simulink model "WindUp"  (R2018b)
settings: Solver=VariableStepAuto  StartTime=0.0  StopTime=100  RelTol=1e-3
settings Model: Creator=Alex  LastModifiedBy=Alex

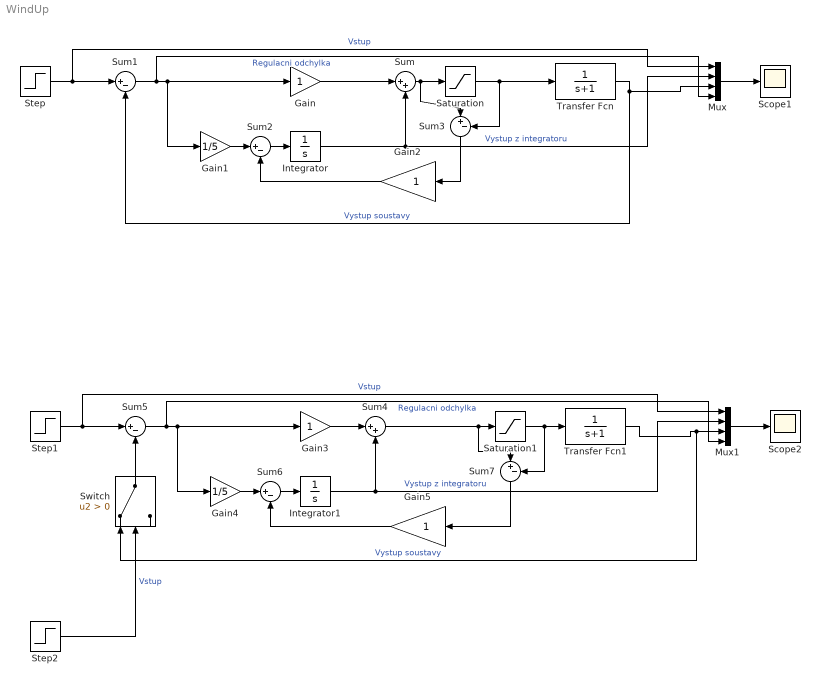
== system WindUp ==
  Gain{,2..3,5} (4 alike) : Gain
  Gain1 : Gain  Gain=1/5
  Gain4 : Gain  Gain=1/5
  Integrator : Integrator
  Integrator1 : Integrator
  Mux : Mux
  Mux1 : Mux
  Saturation : Saturate
  Saturation1 : Saturate
  Scope1 : Scope
  Scope2 : Scope
  Step : Step  Time=30  Before=1  After=0.2  SampleTime=0
  Step1 : Step  Time=30  Before=1  After=0.5  SampleTime=0
  Step2 : Step  Time=30  After=0.5  SampleTime=0
  Sum : Sum  Inputs=|++
  Sum{1..3,5..7} (6 alike) : Sum  Inputs=|+-
  Sum4 : Sum  Inputs=|++
  Switch : Switch  Criteria=u2 > Threshold
  Transfer Fcn : TransferFcn  Denominator=[1 1]
  Transfer Fcn1 : TransferFcn  Denominator=[1 1]
  wires:
  Integrator/1 -> Sum/2, Mux/2  "Vystup z integratoru"
  Gain/1 -> Sum/1
  Sum1/1 -> Mux/4, Gain1/1, Gain/1  "Regulacni odchylka"
  Step/1 -> Mux/1, Sum1/1  "Vstup"
  Sum/1 -> Sum3/1, Saturation/1
  Saturation/1 -> Sum3/2, Transfer Fcn/1
  Transfer Fcn/1 -> Mux/3, Sum1/2  "Vystup soustavy"
  Mux/1 -> Scope1/1
  Gain1/1 -> Sum2/1
  Sum2/1 -> Integrator/1
  Sum3/1 -> Gain2/1
  Gain2/1 -> Sum2/2
  Gain5/1 -> Sum6/2
  Gain3/1 -> Sum4/1
  Integrator1/1 -> Mux1/2, Sum4/2  "Vystup z integratoru"
  Transfer Fcn1/1 -> Switch/1, Mux1/3  "Vystup soustavy"
  Saturation1/1 -> Sum7/2, Transfer Fcn1/1
  Step1/1 -> Mux1/1, Sum5/1  "Vstup"
  Sum5/1 -> Mux1/4, Gain4/1, Gain3/1  "Regulacni odchylka"
  Sum6/1 -> Integrator1/1
  Mux1/1 -> Scope2/1
  Gain4/1 -> Sum6/1
  Sum4/1 -> Sum7/1, Saturation1/1
  Sum7/1 -> Gain5/1
  Switch/1 -> Sum5/2
  Step2/1 -> Switch/2  "Vstup"
